simulink model "Sensores_23"  (R2023b)
settings: Solver=VariableStepAuto  StartTime=0.0  StopTime=10.0  RelTol=1e-3
settings Model: Creator=alber  LastModifiedBy=alber

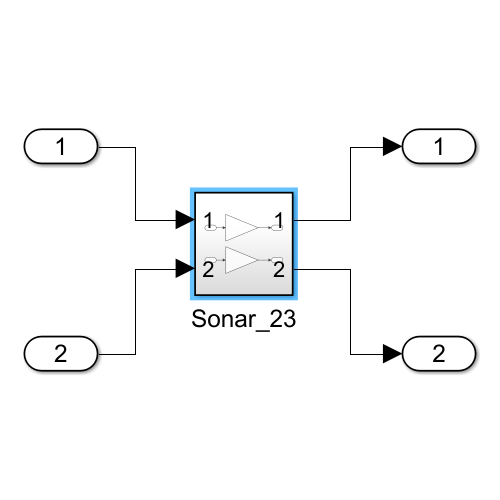
[thumbnail: Simulink's stored preview of the top-level diagram]
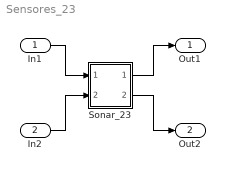
== system Sensores_23 ==
  In1 : Inport
  In2 : Inport  Port=2
  Sonar_23 : Subsystem
  Out1 : Outport
  Out2 : Outport  Port=2
  wires:
  In1/1 -> Sonar_23/1(In1)
  In2/1 -> Sonar_23/2(In2)
  Sonar_23/1(Out1) -> Out1/1
  Sonar_23/2(Out2) -> Out2/1

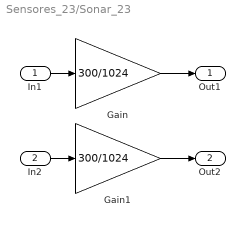
== system Sensores_23/Sonar_23 ==
  In1 : Inport
  In2 : Inport  Port=2
  Gain : Gain  Gain=300/1024
  Gain1 : Gain  Gain=300/1024
  Out1 : Outport
  Out2 : Outport  Port=2
  wires:
  Gain/1 -> Out1/1
  In1/1 -> Gain/1
  In2/1 -> Gain1/1
  Gain1/1 -> Out2/1
